simulink subsystem "ElectromechanicalDynamics"  (R2024b)
settings: Solver=VariableStepAuto  StartTime=0.0  StopTime=10.0  RelTol=1e-3
values from neighbouring files (symbols this model uses):
  Fv1 = Fv + (2 * gbox.N^2 * mot.Kt * mot.Ke/ mot.R)*[1 -1; -1 1]    [Plant_balrob_calculations.m]
  ua2tau = (2 * gbox.N * mot.Kt / mot.R) * [1; -1]    [Plant_balrob_calculations.m]
  x0 = [0; 0; 0; 0]    [A_final_results.m]    (also in Plant_balrob_params.m = [       0,       5*deg2rad,       0,       0])
settings Model: Creator=federico  LastModifiedBy=Riccardo Grosso

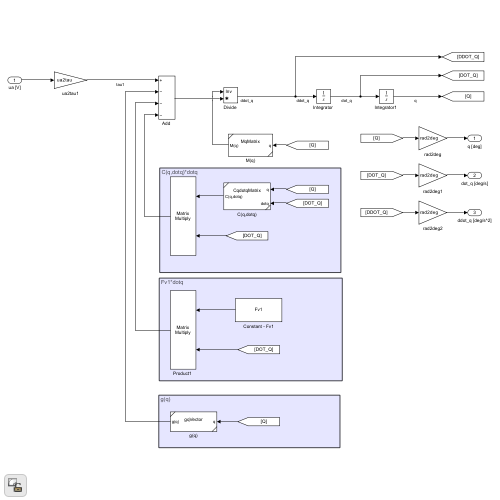
[thumbnail: Simulink's stored preview of the top-level diagram]
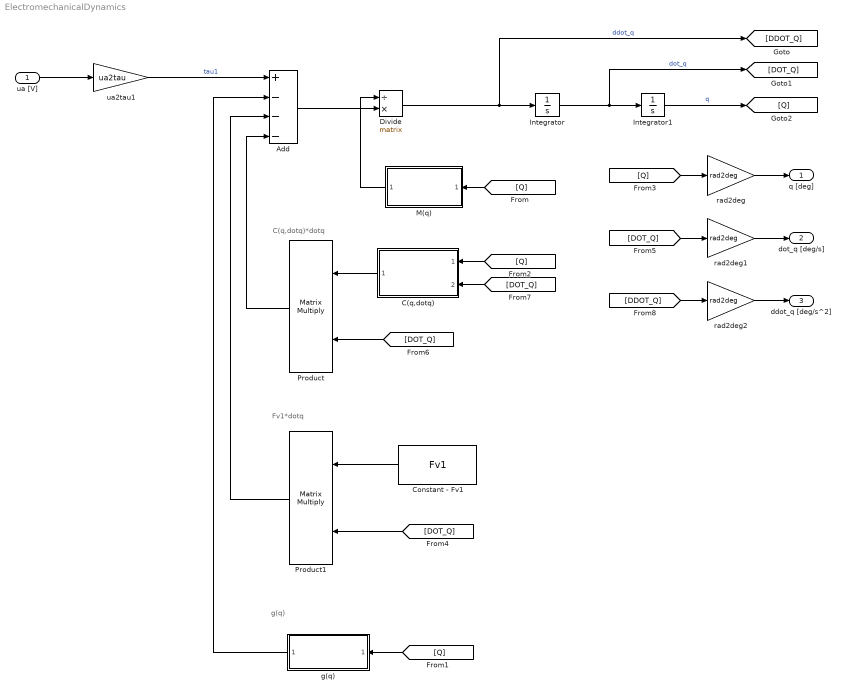
== system ElectromechanicalDynamics ==
  note: g(q)
  note: Fv1*dotq
  note: C(q,dotq)*dotq
  ua [V] : Inport
  "Add " : Sum  Inputs=+---
  C(q,dotq) : Subsystem  ReferencedSubsystem=CqdotqMatrix
  Constant - Fv1 : Constant  Value=Fv1
  "Divide " : Product  Inputs=/*  Multiplication=Matrix(*)
  "Integrator " : Integrator  InitialCondition=x0(3:4,:)
  "Integrator1 " : Integrator  InitialCondition=x0(1:2,:)
  M(q) : Subsystem  ReferencedSubsystem=MqMatrix
  Product : Product  Multiplication=Matrix(*)
  "Product1 " : Product  Multiplication=Matrix(*)
  g(q) : Subsystem  ReferencedSubsystem=gqVector
  rad2deg : Gain  Gain=rad2deg
  rad2deg1 : Gain  Gain=rad2deg
  rad2deg2 : Gain  Gain=rad2deg
  ua2tau1 : Gain  Gain=ua2tau
  q [deg] : Outport
  dot_q [deg/s] : Outport  Port=2
  ddot_q [deg/s^2] : Outport  Port=3
  wires:
  ua [V]/1 -> ua2tau1/1
  ua2tau1/1 -> "Add "/1  "tau1"
  "Add "/1 -> "Divide "/2
  [Q] -> M(q)/1
  "Integrator "/1 -> "Integrator1 "/1, [DOT_Q]  "dot_q"
  "Integrator1 "/1 -> [Q]  "q"
  [Q] -> rad2deg/1
  rad2deg/1 -> q [deg]/1
  [DOT_Q] -> rad2deg1/1
  rad2deg1/1 -> dot_q [deg/s]/1
  [DDOT_Q] -> rad2deg2/1
  rad2deg2/1 -> ddot_q [deg/s^2]/1
  [Q] -> C(q,dotq)/1
  [DOT_Q] -> C(q,dotq)/2
  C(q,dotq)/1 -> Product/1
  [DOT_Q] -> Product/2
  Product/1 -> "Add "/4
  Constant - Fv1/1 -> "Product1 "/1
  [DOT_Q] -> "Product1 "/2
  [Q] -> g(q)/1
  "Product1 "/1 -> "Add "/3
  g(q)/1 -> "Add "/2
  "Divide "/1 -> "Integrator "/1, [DDOT_Q]  "ddot_q"
  M(q)/1 -> "Divide "/1
